simulink model "SimulinkBuses"  (R2018a)
settings: Solver=VariableStepAuto  StartTime=0.0  StopTime=10.0  RelTol=1e-3
settings Model: Creator=Choaib ELMADI  LastModifiedBy=Choaib ELMADI

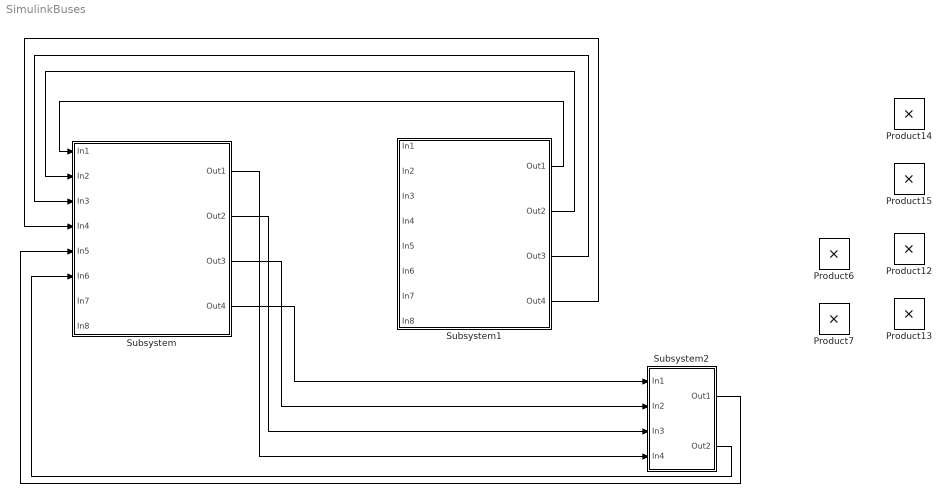
== system SimulinkBuses ==
  Product{6..7,12..15} (6 alike) : Product
  Subsystem : Subsystem
  Subsystem1 : Subsystem
  Subsystem2 : Subsystem
  wires:
  Subsystem1/1(Out1) -> Subsystem/1(In1)
  Subsystem1/2(Out2) -> Subsystem/2(In2)
  Subsystem1/3(Out3) -> Subsystem/3(In3)
  Subsystem1/4(Out4) -> Subsystem/4(In4)
  Subsystem2/1(Out1) -> Subsystem/5(In5)
  Subsystem2/2(Out2) -> Subsystem/6(In6)
  Subsystem/4(Out4) -> Subsystem2/1(In1)
  Subsystem/3(Out3) -> Subsystem2/2(In2)
  Subsystem/2(Out2) -> Subsystem2/3(In3)
  Subsystem/1(Out1) -> Subsystem2/4(In4)

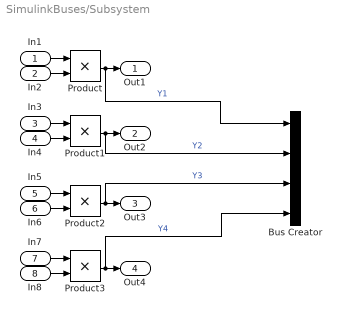
== system SimulinkBuses/Subsystem ==
  In1 : Inport
  In2 : Inport  Port=2
  In3 : Inport  Port=3
  In4 : Inport  Port=4
  In5 : Inport  Port=5
  In6 : Inport  Port=6
  In7 : Inport  Port=7
  In8 : Inport  Port=8
  Bus Creator : BusCreator  Inputs=4
  Product{,1..3} (4 alike) : Product
  Out1 : Outport
  Out2 : Outport  Port=2
  Out3 : Outport  Port=3
  Out4 : Outport  Port=4
  wires:
  In3/1 -> Product1/1
  Product3/1 -> Bus Creator/4, Out4/1  "Y4"
  In4/1 -> Product1/2
  Product1/1 -> Bus Creator/2, Out2/1  "Y2"
  In1/1 -> Product/1
  In6/1 -> Product2/2
  In5/1 -> Product2/1
  In2/1 -> Product/2
  Product/1 -> Bus Creator/1, Out1/1  "Y1"
  In7/1 -> Product3/1
  Product2/1 -> Bus Creator/3, Out3/1  "Y3"
  In8/1 -> Product3/2

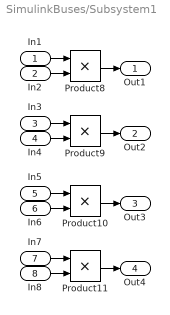
== system SimulinkBuses/Subsystem1 ==
  In1 : Inport
  In2 : Inport  Port=2
  In3 : Inport  Port=3
  In4 : Inport  Port=4
  In5 : Inport  Port=5
  In6 : Inport  Port=6
  In7 : Inport  Port=7
  In8 : Inport  Port=8
  Product{8..11} (4 alike) : Product
  Out1 : Outport
  Out2 : Outport  Port=2
  Out3 : Outport  Port=3
  Out4 : Outport  Port=4
  wires:
  Product9/1 -> Out2/1
  In1/1 -> Product8/1
  Product11/1 -> Out4/1
  In8/1 -> Product11/2
  In7/1 -> Product11/1
  In3/1 -> Product9/1
  In4/1 -> Product9/2
  In2/1 -> Product8/2
  Product8/1 -> Out1/1
  In6/1 -> Product10/2
  Product10/1 -> Out3/1
  In5/1 -> Product10/1

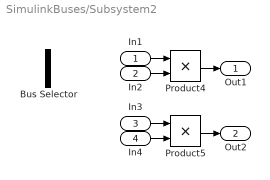
== system SimulinkBuses/Subsystem2 ==
  In1 : Inport
  In2 : Inport  Port=2
  In3 : Inport  Port=3
  In4 : Inport  Port=4
  Bus Selector : BusSelector  OutputSignals=signal1,signal2
  Product4 : Product
  Product5 : Product
  Out1 : Outport
  Out2 : Outport  Port=2
  wires:
  Product5/1 -> Out2/1
  In3/1 -> Product5/1
  Product4/1 -> Out1/1
  In1/1 -> Product4/1
  In2/1 -> Product4/2
  In4/1 -> Product5/2
